simulink model "Lab4_Lead"  (R2016a)
settings: Solver=VariableStepAuto  StartTime=0.0  StopTime=10.0  RelTol=1e-3
settings Model: Creator=jordan  LastModifiedBy=jordan

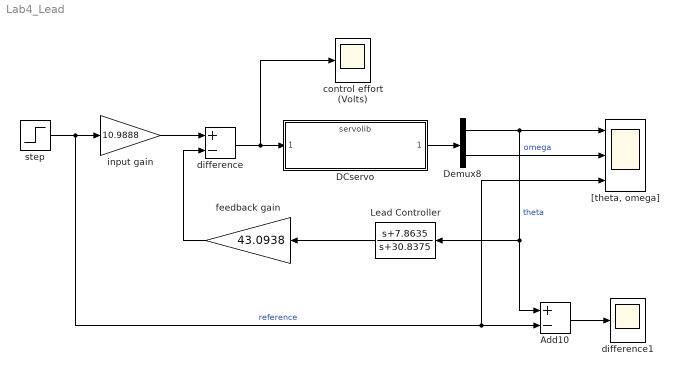
== system Lab4_Lead ==
  Add10 : Sum  Inputs=+-
  DCservo : ModelReference  ModelNameDialog=servolib.slx  SimulationMode=Normal  ModelReferenceVersion=1.77
  Demux8 : Demux  Outputs=2
  Lead Controller : TransferFcn  Numerator=[1 7.8635]  Denominator=[1 30.8375]
  "[theta, omega]" : Scope  NumInputPorts=3
  control effort (Volts) : Scope
  difference : Sum  Inputs=+-
  difference1 : Scope
  feedback gain : Gain  Gain=43.0938
  input gain : Gain  Gain=10.9888
  step : Step  SampleTime=0
  wires:
  Demux8/2 -> "[theta, omega]"/2  "omega"
  step/1 -> "[theta, omega]"/3, Add10/2, input gain/1  "reference"
  feedback gain/1 -> difference/2
  Lead Controller/1 -> feedback gain/1
  input gain/1 -> difference/1
  Add10/1 -> difference1/1
  Demux8/1 -> Add10/1, Lead Controller/1, "[theta, omega]"/1  "theta"
  difference/1 -> control effort (Volts)/1, DCservo/1
  DCservo/1 -> Demux8/1
